simulink model "one"  (R2020b)
settings: Solver=VariableStepAuto  StartTime=0.0  StopTime=10.0  RelTol=1e-3
PreLoadFcn:
  |  M1 = 100;
  |  K1 = 50;
  |  B = 50;
  |  M2=10;
  |  K12=1000;
settings Model: Creator=USER  LastModifiedBy=USER

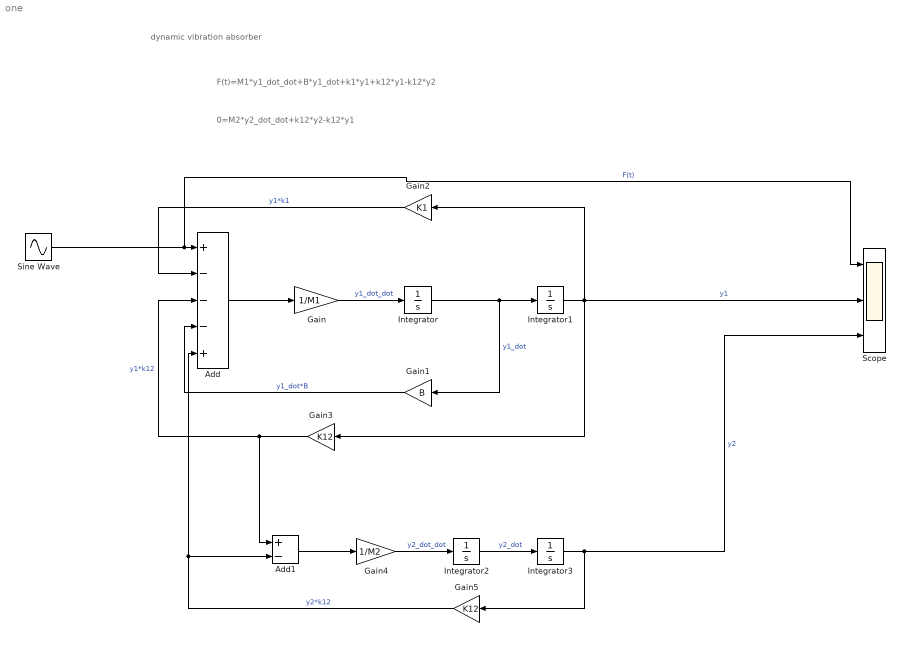
== system one ==
  note: F(t)=M1*y1_dot_dot+B*y1_dot+k1*y1+k12*y1-k12*y2
  note: dynamic vibration absorber
  note: 0=M2*y2_dot_dot+k12*y2-k12*y1
  Add : Sum  Inputs=+---+
  Add1 : Sum  Inputs=+-
  Gain : Gain  Gain=1/M1
  Gain1 : Gain  Gain=B
  Gain2 : Gain  Gain=K1
  Gain3 : Gain  Gain=K12
  Gain4 : Gain  Gain=1/M2
  Gain5 : Gain  Gain=K12
  Integrator{,1..3} (4 alike) : Integrator
  Scope : Scope  NumInputPorts=3
  Sine Wave : Sin  Amplitude=2  Frequency=10  SampleTime=0
  wires:
  Add/1 -> Gain/1
  Gain/1 -> Integrator/1  "y1_dot_dot"
  Integrator/1 -> Integrator1/1, Gain1/1  "y1_dot"
  Integrator1/1 -> Gain2/1, Scope/2, Gain3/1  "y1"
  Gain1/1 -> Add/4  "y1_dot*B"
  Gain2/1 -> Add/2  "y1*k1"
  Gain3/1 -> Add1/1, Add/3  "y1*k12"
  Add1/1 -> Gain4/1
  Gain4/1 -> Integrator2/1  "y2_dot_dot"
  Integrator2/1 -> Integrator3/1  "y2_dot"
  Integrator3/1 -> Scope/3, Gain5/1  "y2"
  Gain5/1 -> Add1/2, Add/5  "y2*k12"
  Sine Wave/1 -> Scope/1, Add/1  "F(t)"
